simulink model "LTR_Simulink"  (R2022a)
settings: Solver=VariableStepAuto  StartTime=0.0  StopTime=3  RelTol=1e-3
values from neighbouring files (symbols this model uses):
  C = eye(5)    [Aircraft_model.m]    (also in LTR.m = [0.5 0.5 0 0)
  Gamma = sysd.B    [Aircraft_model.m]    (also in LTR.m)
  H_I = [-2.113 2.113 0.375 0.375]    [LTR.m]
  K = K_a(:,2:5)    [LTR.m]
  K_I = K_a(:,1)    [LTR.m]
  N_x = [1 -0.2366 ... (first row only)    [LTR.m]
  Phi = sysd.A    [Aircraft_model.m]    (also in LTR.m)
  Rv = [0.0004 0; 0 0.0001]    [LTR.m]
  Rw = [0.0001 0; 0 0.0001]    [LTR.m]
undefined symbols (not defined in the file or in its folder): DiscIntNeverNeededParam, Discrete, Time
libraries: ctrlSharedLib x2
settings Model: Creator=mjwhi  LastModifiedBy=mjwhi

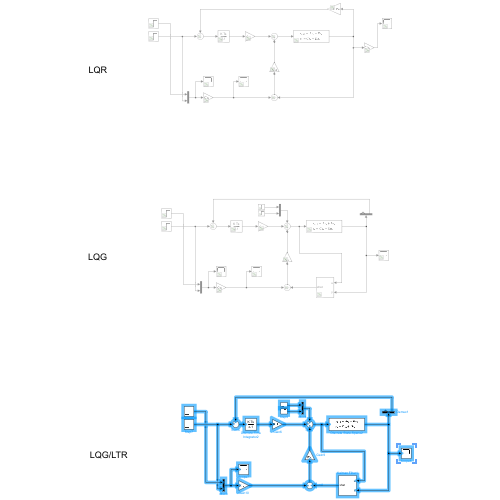
[thumbnail: Simulink's stored preview of the top-level diagram]
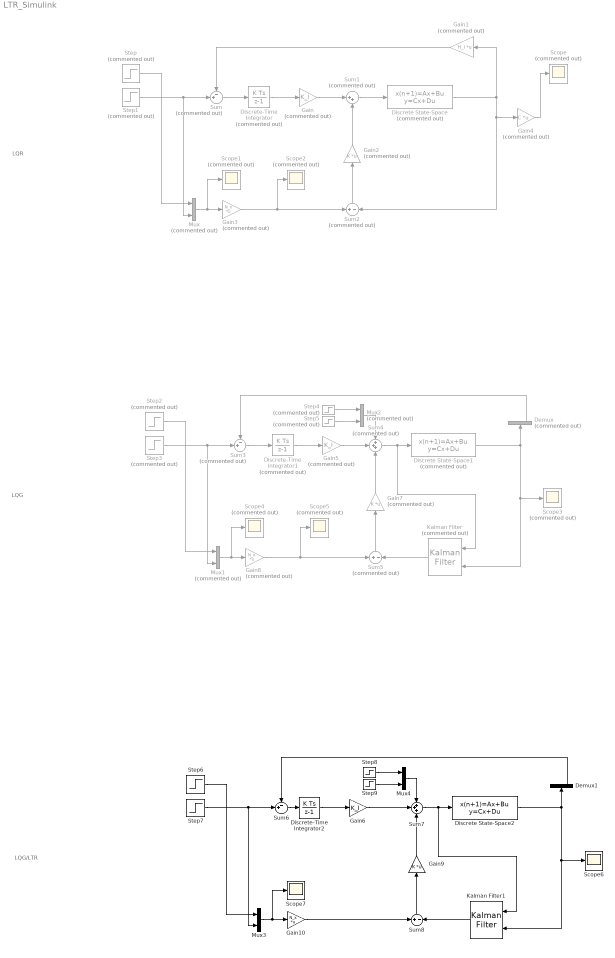
== system LTR_Simulink ==
  note: LQG/LTR
  note: LQG
  note: LQR
  Demux : Demux  Commented=on  Outputs=2
  Demux1 : Demux  Outputs=2
  Discrete State-Space : DiscreteStateSpace  Commented=on  A=Phi  B=Gamma  C=eye(4)  D=zeros(4,2)  SampleTime=0.05
  Discrete State-Space1 : DiscreteStateSpace  Commented=on  A=Phi  B=Gamma  C=C  D=zeros(2,2)  InitialCondition=[100 100 0 100]  SampleTime=0.05
  Discrete State-Space2 : DiscreteStateSpace  A=Phi  B=Gamma  C=C  D=zeros(2,2)  InitialCondition=[100 100 0 100]  SampleTime=0.05
  Discrete-Time Integrator : DiscreteIntegrator  Commented=on  gainval=20  SampleTime=-1  ICPrevOutput=DiscIntNeverNeededParam  ICPrevScaledInput=DiscIntNeverNeededParam
  Discrete-Time Integrator1 : DiscreteIntegrator  Commented=on  gainval=20  SampleTime=-1  ICPrevOutput=DiscIntNeverNeededParam  ICPrevScaledInput=DiscIntNeverNeededParam
  Discrete-Time Integrator2 : DiscreteIntegrator  gainval=sqrt(2)  SampleTime=-1  ICPrevOutput=DiscIntNeverNeededParam  ICPrevScaledInput=DiscIntNeverNeededParam
  Gain : Gain  Commented=on  Gain=K_I
  Gain1 : Gain  Commented=on  Gain=H_I  Multiplication=Matrix(K*u)
  Gain10 : Gain  Gain=N_x  Multiplication=Matrix(K*u)
  Gain2 : Gain  Commented=on  Gain=K  Multiplication=Matrix(K*u)
  Gain3 : Gain  Commented=on  Gain=N_x  Multiplication=Matrix(K*u)
  Gain4 : Gain  Commented=on  Gain=C  Multiplication=Matrix(K*u)
  Gain5 : Gain  Commented=on  Gain=K_I
  Gain6 : Gain  Gain=K_I
  Gain7 : Gain  Commented=on  Gain=K  Multiplication=Matrix(K*u)
  Gain8 : Gain  Commented=on  Gain=N_x  Multiplication=Matrix(K*u)
  Gain9 : Gain  Gain=K  Multiplication=Matrix(K*u)
  Kalman Filter : ctrlSharedLib/Kalman Filter  Commented=on  TimeDomain=Discrete-Time  UseCurrentEstimator=on  ModelSource=Individual A, B, C, D matrices  ModelSourceVariable=ss(0.95,1,1,0,1)  A=Phi  B=Gamma  C=C  D=zeros(2,2)  NumberOfStates=1  NumberOfInputs=1  NumberOfOutputs=1  InitialEstimateSource=Dialog  X0=0  P0=10  UseK=off  UseGH=off  NumberOfProcessNoiseInputs=1  G=1  TimeInvariantG=on  H=0  TimeInvariantH=on  Q=Gamma*Rv*Gamma'  TimeInvariantQ=on  R=Rw  TimeInvariantR=on  N=0  TimeInvariantN=on  AddInputPort=on  AddEnablePort=off  OutputEstimatedY=off  OutputP=off  Ts=-1
  Kalman Filter1 : ctrlSharedLib/Kalman Filter  TimeDomain=Discrete-Time  UseCurrentEstimator=on  ModelSource=Individual A, B, C, D matrices  ModelSourceVariable=ss(0.95,1,1,0,1)  A=Phi  B=Gamma  C=C  D=zeros(2,2)  NumberOfStates=1  NumberOfInputs=1  NumberOfOutputs=1  InitialEstimateSource=Dialog  X0=0  P0=10  UseK=off  UseGH=off  NumberOfProcessNoiseInputs=1  G=1  TimeInvariantG=on  H=0  TimeInvariantH=on  Q=Gamma*Rv*Gamma'  TimeInvariantQ=on  R=Rw  TimeInvariantR=on  N=0  TimeInvariantN=on  AddInputPort=on  AddEnablePort=off  OutputEstimatedY=off  OutputP=off  Ts=-1
  Mux : Mux  Commented=on  Inputs=2
  Mux1 : Mux  Commented=on  Inputs=2
  Mux2 : Mux  Commented=on  Inputs=2
  Mux3 : Mux  Inputs=2
  Mux4 : Mux  Inputs=2
  Scope{,1..5} (6 alike) : Scope  Commented=on
  Scope6 : Scope
  Scope7 : Scope
  Step : Step  Commented=on  Time=0  SampleTime=0.05
  Step1 : Step  Commented=on  Time=0  After=2  SampleTime=0
  Step2 : Step  Commented=on  Time=0  SampleTime=0.05
  Step3 : Step  Commented=on  Time=0  After=2  SampleTime=0.05
  Step4 : Step  Commented=on  Time=1.5  After=0.01  SampleTime=0.05
  Step5 : Step  Commented=on  After=0  SampleTime=0.05
  Step6 : Step  Time=0  SampleTime=0.05
  Step7 : Step  Time=0  After=2  SampleTime=0.05
  Step8 : Step  Time=1.5  After=0.01  SampleTime=0.05
  Step9 : Step  After=0  SampleTime=0.05
  Sum : Sum  Commented=on  Inputs=-+|
  Sum1 : Sum  Commented=on  Inputs=|++
  Sum2 : Sum  Commented=on  Inputs=+|-
  Sum3 : Sum  Commented=on  Inputs=-+|
  Sum4 : Sum  Commented=on  Inputs=+++
  Sum5 : Sum  Commented=on  Inputs=+|-
  Sum6 : Sum  Inputs=-+|
  Sum7 : Sum  Inputs=+++
  Sum8 : Sum  Inputs=+|-
  wires:
  Step/1 -> Mux/1
  Step1/1 -> Mux/2, Sum/2
  Sum/1 -> Discrete-Time Integrator/1
  Gain/1 -> Sum1/1
  Sum1/1 -> Discrete State-Space/1
  Discrete State-Space/1 -> Gain4/1, Sum2/2, Gain1/1
  Gain1/1 -> Sum/1
  Sum2/1 -> Gain2/1
  Gain2/1 -> Sum1/2
  Mux/1 -> Scope1/1, Gain3/1
  Gain3/1 -> Scope2/1, Sum2/1
  Discrete-Time Integrator/1 -> Gain/1
  Gain4/1 -> Scope/1
  Gain7/1 -> Sum4/3
  Sum5/1 -> Gain7/1
  Discrete-Time Integrator1/1 -> Gain5/1
  Gain5/1 -> Sum4/2
  Discrete State-Space1/1 -> Scope3/1, Kalman Filter/2, Demux/1
  Sum3/1 -> Discrete-Time Integrator1/1
  Step2/1 -> Mux1/1
  Demux/2 -> Sum3/1
  Sum4/1 -> Kalman Filter/1, Discrete State-Space1/1
  Step3/1 -> Mux1/2, Sum3/2
  Gain8/1 -> Scope5/1, Sum5/1
  Mux1/1 -> Scope4/1, Gain8/1
  Kalman Filter/1 -> Sum5/2
  Step4/1 -> Mux2/1
  Step5/1 -> Mux2/2
  Mux2/1 -> Sum4/1
  Demux1/2 -> Sum6/1
  Gain6/1 -> Sum7/2
  Mux4/1 -> Sum7/1
  Gain9/1 -> Sum7/3
  Mux3/1 -> Scope7/1, Gain10/1
  Gain10/1 -> Sum8/1
  Step6/1 -> Mux3/1
  Discrete-Time Integrator2/1 -> Gain6/1
  Discrete State-Space2/1 -> Scope6/1, Kalman Filter1/2, Demux1/1
  Step7/1 -> Mux3/2, Sum6/2
  Sum7/1 -> Kalman Filter1/1, Discrete State-Space2/1
  Sum8/1 -> Gain9/1
  Step8/1 -> Mux4/1
  Sum6/1 -> Discrete-Time Integrator2/1
  Step9/1 -> Mux4/2
  Kalman Filter1/1 -> Sum8/2
